simulink model "l7sim3"  (R2022b)
settings: Solver=VariableStepAuto  StartTime=0.0  StopTime=10.0  RelTol=1e-3
values from neighbouring files (symbols this model uses):
  A = [0 1; -g/l -b/(m*l^2)]    [l2p41.m]    (also in l5ex3.m = fscanf(fileID, '; l7ex1.m = [0.5 -2; -0.5 -0.3]; l7ex2.m = [1 -4 4; 1 0 0; 0 1 0]; l7ex2v2.m = [1 -4 4; 1 0 0; 0 1 0])
  B = [0; 1/(m*l^2)]    [l2p41.m]    (also in l7ex1.m = [1;0]; l7ex2.m = [1; 0; 0]; l7ex2v2.m = [1; 0; 0]; l7ex3.m = [1; 0; 0])
  C = 0.6    [ex3l2.m]    (also in l2p41.m = [1 0]; l7ex1.m = eye (2); l7ex2.m = [0 1 -1]; l7ex2v2.m = eye ( 3 ))
  C2 = eye(3)    [l7ex3.m]
  D = 0    [l2p41.m]    (also in l7ex1.m = [0;0]; l7ex2.m = [0]; l7ex2v2.m = [0;0;0]; l7ex3.m = [0;0;0])
  K = 1    [ex2l3.m]    (also in ex3l2.m = 3; l3ex7.m = rltool(G); l7ex1.m = place (A, B, [-1 -2]); l7ex2.m = place (A, B, [-1 -2]))
  N = 1/(C*inv(A-B*K)*B)    [l7ex3.m]
settings Model: Creator=gokuz  LastModifiedBy=gokuz

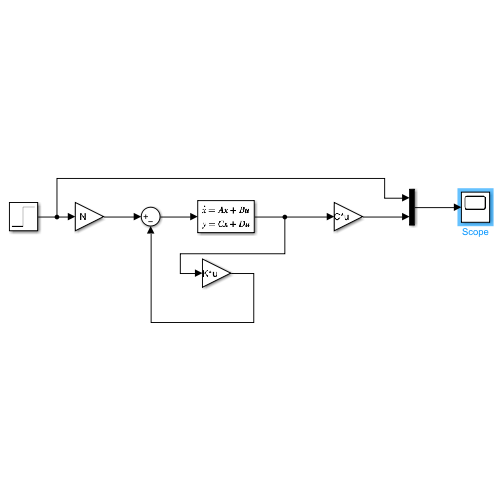
[thumbnail: Simulink's stored preview of the top-level diagram]
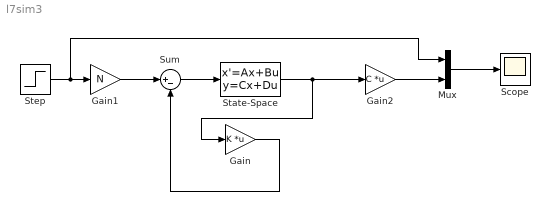
== system l7sim3 ==
  Gain : Gain  Gain=K  Multiplication=Matrix(K*u)
  Gain1 : Gain  Gain=N
  Gain2 : Gain  Gain=C  Multiplication=Matrix(K*u)
  Mux : Mux  Inputs=2
  Scope : Scope
  State-Space : StateSpace  A=A  B=B  C=C2  D=D  InitialCondition=0  ParameterTunability=Unconstrained
  Step : Step  SampleTime=0
  Sum : Sum  Inputs=|+-
  wires:
  Step/1 -> Mux/1, Gain1/1
  Gain1/1 -> Sum/1
  Sum/1 -> State-Space/1
  State-Space/1 -> Gain/1, Gain2/1
  Gain/1 -> Sum/2
  Gain2/1 -> Mux/2
  Mux/1 -> Scope/1
